simulink model "pendulum_model"  (R2015a)
settings: Solver=ode8  StartTime=0.0  StopTime=params.tf  FixedStep=1e-2  RelTol=1e-10  AbsTol=1e-10
values from neighbouring files (symbols this model uses):
  params = [g, m0, b0,                m1, I1, b1, L1, L1_cg,                Kt, Ke, Ra, Vcc, D]    [load_params.m]    (also in s_pendulum.m = [])
libraries: aerolibutil x1
settings Model: Creator=BPeixoto  LastModifiedBy=BPeixoto
settings SolverCC: ShapePreserveControl=EnableAll

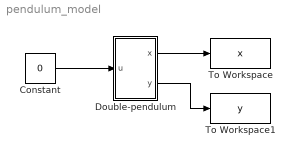
== system pendulum_model ==
  Constant : Constant  Value=0
  Double-pendulum : Subsystem
  To Workspace : ToWorkspace  VariableName=x  SaveFormat=Structure With Time  SampleTime=-1
  To Workspace1 : ToWorkspace  VariableName=y  SaveFormat=Structure With Time  SampleTime=-1
  wires:
  Double-pendulum/1(x) -> To Workspace/1
  Double-pendulum/2(y) -> To Workspace1/1
  Constant/1 -> Double-pendulum/1(u)

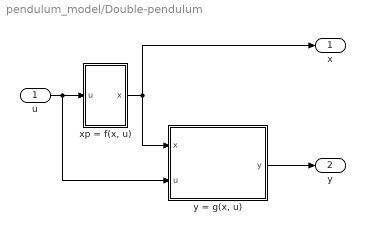
== system pendulum_model/Double-pendulum ==
  u : Inport
  "xp = f(x, u)" : Subsystem
  "y = g(x, u)" : MATLAB Function  TreatAsAtomicUnit=on
  x : Outport
  y : Outport  Port=2
  wires:
  u/1 -> "y = g(x, u)"/2(u), "xp = f(x, u)"/1(u)
  "y = g(x, u)"/1(y) -> y/1
  "xp = f(x, u)"/1(x) -> x/1, "y = g(x, u)"/1(x)

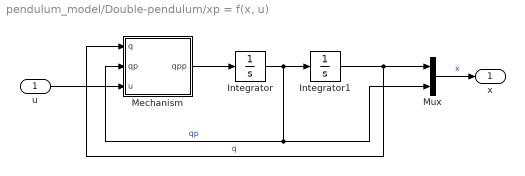
== system pendulum_model/Double-pendulum/xp = f(x, u) ==
  u : Inport
  Integrator : Integrator  InitialCondition=params.qp0
  Integrator1 : Integrator  InitialCondition=params.q0
  Mechanism : Subsystem
  Mux : Mux  Inputs=2
  x : Outport
  wires:
  Mux/1 -> x/1  "x"
  u/1 -> Mechanism/3(u)
  Integrator/1 -> Integrator1/1, Mechanism/2(qp), Mux/2  "qp"
  Mechanism/1(qpp) -> Integrator/1
  Integrator1/1 -> Mux/1, Mechanism/1(q)  "q"

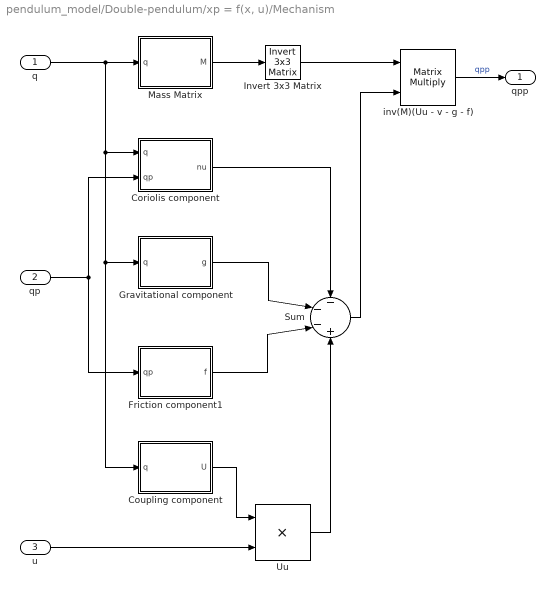
== system pendulum_model/Double-pendulum/xp = f(x, u)/Mechanism ==
  q : Inport
  qp : Inport  Port=2
  u : Inport  Port=3
  Coriolis component : MATLAB Function  TreatAsAtomicUnit=on
  Coupling component : MATLAB Function  TreatAsAtomicUnit=on
  Friction component1 : MATLAB Function  TreatAsAtomicUnit=on
  Gravitational component : MATLAB Function  TreatAsAtomicUnit=on
  Invert 3x3 Matrix : aerolibutil/Invert  3x3 Matrix
  Mass Matrix : MATLAB Function  TreatAsAtomicUnit=on
  Sum : Sum  Inputs=-|-|-|+
  Uu : Product
  inv(M)(Uu - v - g - f) : Product  Multiplication=Matrix(*)
  qpp : Outport
  wires:
  Mass Matrix/1(M) -> Invert 3x3 Matrix/1
  Coriolis component/1(nu) -> Sum/1
  qp/1 -> Coriolis component/2(qp), Friction component1/1(qp)
  q/1 -> Coupling component/1(q), Gravitational component/1(q), Coriolis component/1(q), Mass Matrix/1(q)
  Gravitational component/1(g) -> Sum/2
  Friction component1/1(f) -> Sum/3
  Invert 3x3 Matrix/1 -> inv(M)(Uu - v - g - f)/1
  Sum/1 -> inv(M)(Uu - v - g - f)/2
  inv(M)(Uu - v - g - f)/1 -> qpp/1  "qpp"
  Coupling component/1(U) -> Uu/1
  u/1 -> Uu/2
  Uu/1 -> Sum/4

== matlab function pendulum_model/Double-pendulum/xp = f(x, u)/Mechanism/Coriolis component ==
  data: q input; qp input; nu output; params parameter
function nu = corvec(q, qp, params)
    % Coriolis 'vector
    nu = zeros(3, 1);
    
    % Coupled mass matrix
    nu(1) = -params.m2*params.L2_cg*sin(q(2) + q(3))*(qp(2) + qp(3)^2 ...
            -(params.m2*params.L1 + params.m1*params.L1_cg)*sin(q(2))*qp(3)^2);
    nu(2) = -params.m2*qp(3)*(2*qp(2) + qp(3))*params.L2_cg*params.L1*sin(q(3));
    nu(3) = params.m2*(qp(2)^2)*params.L2_cg*params.L1*sin(q(3));
end

== matlab function pendulum_model/Double-pendulum/xp = f(x, u)/Mechanism/Mass Matrix ==
  data: q input; M output; params parameter
function M = mmatrix(q, params)
    % Mass matrix
    M = zeros(3, 3);
    
    % Coupled mass matrix
    M(1,1) = params.m0 + params.m1 + params.m2;
    
    M(2,2) = params.m2*params.L1^2 + params.m1*params.L1_cg^2 +...
             params.m2*params.L2_cg^2 + ...
             params.I1 + params.I2 + 2*params.m2*params.L1*params.L2_cg*cos(q(3));
    
    M(3,3) = params.m2*params.L2_cg^2 + params.I2;
         
    M(1,2) = params.m2*params.L2_cg*cos(q(2) + q(3)) + ...
            (params.m2*params.L1 + params.m1*params.L1_cg)*cos(q(2));
    
    M(1,3) = params.m2*params.L2_cg*cos(q(2) + q(3));
    
    M(2,3) = params.m2*params.L2_cg^2 + params.I2 + ...
             params.m2*params.L1*params.L2_cg*cos(q(3));
    
    M(2,1) = M(1,2);
    M(3,1) = M(1,3);
    M(3,2) = M(2,3);
end

== matlab function pendulum_model/Double-pendulum/xp = f(x, u)/Mechanism/Gravitational component ==
  data: q input; g output; params parameter
function g = gvec(q, params)
    % Gravitational component
    g = zeros(3, 1);
    
    % Coupled mass matrix
    g(1) = 0;
    g(2) = params.m2*params.g*(params.L1*sin(q(2)) + ...
           params.L2_cg*sin(q(2) + q(3))) + ...
           params.m1*params.L1_cg*params.g*sin(q(2));
    g(3) = params.m2*params.g*params.L2_cg*sin(q(2) + q(3));
end

== matlab function pendulum_model/Double-pendulum/xp = f(x, u)/Mechanism/Friction component1 ==
  data: qp input; f output; params parameter
function f = fvec(qp, params)
    % Friction vector
    f = zeros(3, 1);
    
    % Coupled mass matrix
    f(1) = params.b0*qp(1);
    f(2) = params.b1*qp(2);
    f(3) = params.b2*qp(3);
end

== matlab function pendulum_model/Double-pendulum/xp = f(x, u)/Mechanism/Coupling component ==
  data: q input; U output
function U = Uvec(q)
    U = [1; 0; 0];
end

== matlab function pendulum_model/Double-pendulum/y = g(x, u) ==
  data: x input; y output; u input
function y = system_output(x, u)
    y = [x(1); x(2); x(3)];
end
